simulink model "DatcomForceMoment"  (Simulink 8.8)
settings: Solver=FixedStepDiscrete  StartTime=0.0  StopTime=0.1  FixedStep=.1  RelTol=1e-3
values from neighbouring files (symbols this model uses):
  nfs = PlaneData('SI')    [AFDSimInit.m]    (also in AFDSimInitDatcom.m; TransferFunction.m = PlaneData('Imperial'))
undefined symbols (not defined in the file or in its folder): datcom, Newton, Raphson, sigbuilder_block
libraries: aerolibutil x12, aerolibtransform2 x1, aerolibasang x1
(part 1 of 2)
settings Model: Creator=AHKh  LastModifiedBy=AHKh
settings DataIOCC: LimitDataPoints=off  SaveFormat=Dataset  SignalLoggingSaveFormat=Dataset  SignalLogging=off  DSMLogging=off  SaveTime=off
settings OptimizationCC: LifeSpan=auto
settings DebuggingCC: UnderspecifiedInitializationDetection=Simplified  MergeDetectMultiDrivingBlocksExec=error  FcnCallInpInsideContextMsg=error  StateNameClashWarn=none  SFUnexpectedBacktrackingDiag=error  SFNoUnconditionalDefaultTransitionDiag=error  SFExecutionAtInitializationDiag=warning
settings HardwareCC: ProdBitPerPointer=64  ProdBitPerSizeT=64  ProdBitPerPtrDiffT=64  ProdLargestAtomicFloat=Float  ProdIntDivRoundTo=Zero  ProdEndianess=LittleEndian  ProdWordSize=64  ProdHWDeviceType=Intel->x86-64 (Windows64)
settings ModelReferenceCC: PropagateSignalLabelsOutOfModel=on
settings GRTTargetCC: TargetLangStandard=C99 (ISO)  GeneratePreprocessorConditionals=Use local settings  CombineOutputUpdateFcns=on  GRTInterface=off
settings ConfigComp: CovMetricSettings=dwe  CovHtmlReporting=off  CovSaveCumulativeToWorkspaceVar=off  CovSaveSingleToWorkspaceVar=off  CovExternalEMLEnable=on

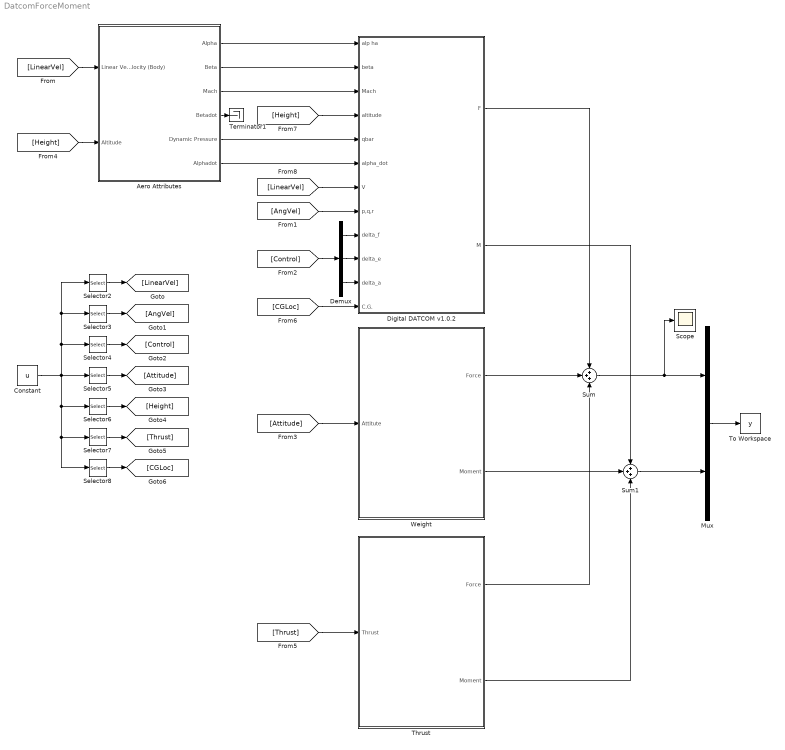
== system DatcomForceMoment ==
  Aero Attributes : Subsystem
  Constant : Constant  Value=u
  Demux : Demux  Outputs=3
  Digital DATCOM v1.0.2 : Subsystem  mask(DATCOM Aerodynamic Forces and Moments Estimation){datcom=datcom}
      mask prompts: datcom "Datcom Structure"
      mask Display:
      | port_label('input',1,'\alpha (rad)','texmode','on');
      | port_label('input',2,'\beta (rad)','texmode','on');
      | port_label('input',3,'Mach','texmode','on');
      | port_label('input',4,'h (m)','texmode','on');
      | port_label('input',5,'q_{bar}','texmode','on');
      | port_label('input',6,'d\alpha/dt (rad/s)','texmode','on');
      | port_label('input',7,'V_{body} m/s','texmode','on');
      | port_label('input',8,'\omega (rad/s)','texmode','on');
      | port_label('input',9,'\delta_F (rad)','texmode','on');
      | port_label('input',10,'\delta_E (rad)','texmode','on');
      | port_label('input',11,'\delta_A (rad)','texmode','on');
      | port_label('input',12,'C.G. (m)','texmode','on');
      | port_label('output',1,'F_{body} (N)','texmode','on');
      | port_label('output',2,'M_{body} (N.m)','texmode','on');
  Mux : Mux  Inputs=2
  Scope : Scope
  Selector2 : Selector  InputPortWidth=17  IndexOptions=Index vector (dialog)  Indices=[1:3]  OutputSizes=1
  Selector3 : Selector  InputPortWidth=17  IndexOptions=Index vector (dialog)  Indices=[4:6]  OutputSizes=1
  Selector4 : Selector  InputPortWidth=17  IndexOptions=Index vector (dialog)  Indices=[7:9]  OutputSizes=1
  Selector5 : Selector  InputPortWidth=17  IndexOptions=Index vector (dialog)  Indices=[10:12]  OutputSizes=1
  Selector6 : Selector  InputPortWidth=17  IndexOptions=Index vector (dialog)  Indices=[13]  OutputSizes=1
  Selector7 : Selector  InputPortWidth=17  IndexOptions=Index vector (dialog)  Indices=[14]  OutputSizes=1
  Selector8 : Selector  InputPortWidth=17  IndexOptions=Index vector (dialog)  Indices=[15:17]  OutputSizes=1
  Sum : Sum  Inputs=+++
  Sum1 : Sum  Inputs=+++
  Terminator1 : Terminator
  "Thrust " : Subsystem
  To Workspace : ToWorkspace  VariableName=y  SampleTime=-1
  Weight : Subsystem
  wires:
  [Height] -> Aero Attributes/2(Altitude)
  [LinearVel] -> Aero Attributes/1(Linear Velocity (Body))
  Aero Attributes/4(Betadot) -> Terminator1/1
  [AngVel] -> Digital DATCOM v1.0.2/8(p,q,r)
  [Height] -> Digital DATCOM v1.0.2/4(altitude)
  [Control] -> Demux/1
  Demux/1 -> Digital DATCOM v1.0.2/9(delta_f)
  Demux/2 -> Digital DATCOM v1.0.2/10(delta_e)
  Demux/3 -> Digital DATCOM v1.0.2/11(delta_a)
  [LinearVel] -> Digital DATCOM v1.0.2/7(V)
  Aero Attributes/1(Alpha) -> Digital DATCOM v1.0.2/1(alp ha)
  Aero Attributes/2(Beta) -> Digital DATCOM v1.0.2/2(beta)
  Aero Attributes/5(Dynamic Pressure) -> Digital DATCOM v1.0.2/5(qbar)
  Aero Attributes/3(Mach) -> Digital DATCOM v1.0.2/3(Mach)
  Aero Attributes/6(Alphadot) -> Digital DATCOM v1.0.2/6(alpha_dot)
  [Attitude] -> Weight/1(Attitute)
  Digital DATCOM v1.0.2/1(F) -> Sum/1
  Weight/1(Force) -> Sum/2
  "Thrust "/1(Force) -> Sum/3
  Sum/1 -> Scope/1, Mux/1
  Weight/2(Moment) -> Sum1/2
  Digital DATCOM v1.0.2/2(M) -> Sum1/1
  "Thrust "/2(Moment) -> Sum1/3
  Sum1/1 -> Mux/2
  [CGLoc] -> Digital DATCOM v1.0.2/12(C.G.)
  [Thrust] -> "Thrust "/1(Thrust)
  Constant/1 -> Selector6/1, Selector8/1, Selector7/1, Selector2/1, Selector3/1, Selector4/1, Selector5/1
  Selector2/1 -> [LinearVel]
  Selector3/1 -> [AngVel]
  Selector4/1 -> [Control]
  Selector5/1 -> [Attitude]
  Selector6/1 -> [Height]
  Selector7/1 -> [Thrust]
  Selector8/1 -> [CGLoc]
  Mux/1 -> To Workspace/1

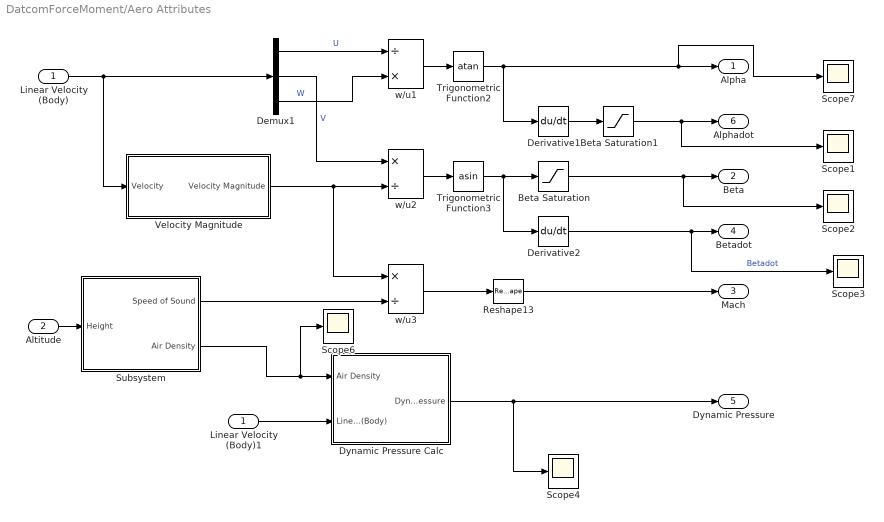
== system DatcomForceMoment/Aero Attributes ==
  Linear Velocity (Body) : Inport  PortDimensions=[3,1]
  Altitude : Inport  Port=2
  Beta Saturation : Saturate  UpperLimit=5*pi/11  LowerLimit=-5*pi/11
  Beta Saturation1 : Saturate  UpperLimit=1  LowerLimit=-1
  Demux1 : Demux  Outputs=3
  Derivative1 : Derivative
  Derivative2 : Derivative
  Dynamic Pressure Calc : Subsystem
  Linear Velocity (Body)1 : InportShadow  PortDimensions=[3,1]
  Reshape13 : Reshape
  Scope{1..4,6..7} (6 alike) : Scope
  Subsystem : Subsystem
  Trigonometric Function2 : Trigonometry  Operator=atan
  Trigonometric Function3 : Trigonometry  Operator=asin
  Velocity Magnitude : Subsystem
  w/u1 : Product  Inputs=/*  SaturateOnIntegerOverflow=on  InputSameDT=on  OutDataTypeStr=Inherit: Same as first input
  w/u2 : Product  Inputs=*/  SaturateOnIntegerOverflow=on  InputSameDT=on  OutDataTypeStr=Inherit: Same as first input
  w/u3 : Product  Inputs=*/  SaturateOnIntegerOverflow=on  InputSameDT=on  OutDataTypeStr=Inherit: Same as first input
  Alpha : Outport
  Beta : Outport  Port=2
  Mach : Outport  Port=3
  Betadot : Outport  Port=4
  Dynamic Pressure : Outport  Port=5
  Alphadot : Outport  Port=6
  wires:
  Beta Saturation1/1 -> Alphadot/1, Scope1/1
  Subsystem/2(Air Density) -> Scope6/1, Dynamic Pressure Calc/1(Air Density)
  Subsystem/1(Speed of Sound) -> w/u3/2
  Velocity Magnitude/1(Velocity Magnitude) -> w/u3/1, w/u2/2
  Reshape13/1 -> Mach/1
  Derivative2/1 -> Betadot/1, Scope3/1  "Betadot"
  Beta Saturation/1 -> Beta/1, Scope2/1
  Derivative1/1 -> Beta Saturation1/1
  Dynamic Pressure Calc/1(Dynamic Pressure) -> Scope4/1, Dynamic Pressure/1
  Linear Velocity (Body)1/1 -> Dynamic Pressure Calc/2(Linear Velocity (Body))
  Altitude/1 -> Subsystem/1(Height)
  w/u3/1 -> Reshape13/1
  Trigonometric Function3/1 -> Beta Saturation/1, Derivative2/1
  Trigonometric Function2/1 -> Derivative1/1, Alpha/1, Scope7/1
  w/u2/1 -> Trigonometric Function3/1
  w/u1/1 -> Trigonometric Function2/1
  Demux1/3 -> w/u1/2  "W"
  Demux1/2 -> w/u2/1  "V"
  Demux1/1 -> w/u1/1  "U"
  Linear Velocity (Body)/1 -> Velocity Magnitude/1(Velocity), Demux1/1

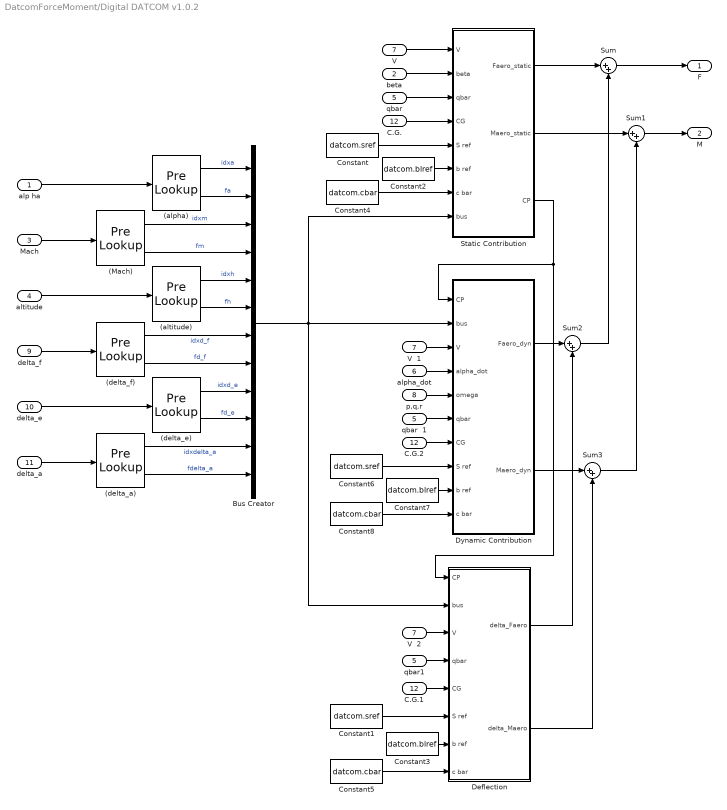
== system DatcomForceMoment/Digital DATCOM v1.0.2 ==
  alp ha : Inport  Unit=rad
  beta : Inport  Port=2  Unit=rad
  Mach : Inport  Port=3  Unit=1
  altitude : Inport  Port=4  Unit=m
  qbar : Inport  Port=5  Unit=Pa
  alpha_dot : Inport  Port=6  Unit=rad/s
  V : Inport  Port=7  Unit=m/s
  p,q,r : Inport  Port=8  Unit=rad/s
  delta_f : Inport  Port=9  Unit=rad
  delta_e : Inport  Port=10  Unit=rad
  delta_a : Inport  Port=11  Unit=rad
  C.G. : Inport  Port=12  Unit=m
  (Mach) : PreLookup  BreakpointsData=datcom.mach  BeginIndexSearchUsingPreviousIndexResult=on  IndexDataTypeStr=int32  FractionDataTypeStr=double
  (alpha) : PreLookup  BreakpointsData=datcom.alpha  BeginIndexSearchUsingPreviousIndexResult=on  IndexDataTypeStr=int32  FractionDataTypeStr=double
  (altitude) : PreLookup  BreakpointsData=datcom.alt  BeginIndexSearchUsingPreviousIndexResult=on  IndexDataTypeStr=int32  FractionDataTypeStr=double
  (delta_a) : PreLookup  BreakpointsData=datcom.deltal-datcom.deltar  BeginIndexSearchUsingPreviousIndexResult=on  IndexDataTypeStr=int32  FractionDataTypeStr=double
  (delta_e) : PreLookup  BreakpointsData=datcom.delta  BeginIndexSearchUsingPreviousIndexResult=on  IndexDataTypeStr=int32  FractionDataTypeStr=double
  (delta_f) : PreLookup  BreakpointsData=datcom.delta  BeginIndexSearchUsingPreviousIndexResult=on  IndexDataTypeStr=int32  FractionDataTypeStr=double
  Bus Creator : BusCreator  Inputs=12
  C.G.1 : InportShadow  Port=12  Unit=m
  C.G.2 : InportShadow  Port=12  Unit=m
  Constant : Constant  Value=datcom.sref
  Constant1 : Constant  Value=datcom.sref
  Constant2 : Constant  Value=datcom.blref
  Constant3 : Constant  Value=datcom.blref
  Constant4 : Constant  Value=datcom.cbar
  Constant5 : Constant  Value=datcom.cbar
  Constant6 : Constant  Value=datcom.sref
  Constant7 : Constant  Value=datcom.blref
  Constant8 : Constant  Value=datcom.cbar
  Deflection : Subsystem
  Dynamic Contribution : Subsystem
  Static Contribution : Subsystem
  Sum{,1..3} (4 alike) : Sum  Inputs=|++
  V  1 : InportShadow  Port=7  Unit=m/s
  V  2 : InportShadow  Port=7  Unit=m/s
  qbar  1 : InportShadow  Port=5  Unit=Pa
  qbar1 : InportShadow  Port=5  Unit=Pa
  F : Outport  Unit=N
  M : Outport  Port=2  Unit=N*m
  wires:
  Constant8/1 -> Dynamic Contribution/10(c bar)
  Constant6/1 -> Dynamic Contribution/8(S ref)
  Constant7/1 -> Dynamic Contribution/9(b ref)
  C.G.2/1 -> Dynamic Contribution/7(CG)
  Constant4/1 -> Static Contribution/7(c bar)
  Constant5/1 -> Deflection/8(c bar)
  Constant3/1 -> Deflection/7(b ref)
  Constant2/1 -> Static Contribution/6(b ref)
  Constant1/1 -> Deflection/6(S ref)
  Constant/1 -> Static Contribution/5(S ref)
  C.G.1/1 -> Deflection/5(CG)
  C.G./1 -> Static Contribution/4(CG)
  Deflection/2(delta_Maero) -> Sum3/2
  Deflection/1(delta_Faero) -> Sum2/2
  Sum3/1 -> Sum1/2
  Sum2/1 -> Sum/2
  qbar1/1 -> Deflection/4(qbar)
  V  2/1 -> Deflection/3("V ")
  (delta_a)/2 -> Bus Creator/12  "fdelta_a"
  (delta_a)/1 -> Bus Creator/11  "idxdelta_a"
  (delta_e)/2 -> Bus Creator/10  "fd_e"
  (delta_e)/1 -> Bus Creator/9  "idxd_e"
  V/1 -> Static Contribution/1("V ")
  V  1/1 -> Dynamic Contribution/3(V)
  qbar/1 -> Static Contribution/3(qbar)
  beta/1 -> Static Contribution/2(beta)
  (alpha)/2 -> Bus Creator/2  "fa"
  (Mach)/2 -> Bus Creator/4  "fm"
  (altitude)/2 -> Bus Creator/6  "fh"
  (altitude)/1 -> Bus Creator/5  "idxh"
  (delta_f)/2 -> Bus Creator/8  "fd_f"
  (delta_f)/1 -> Bus Creator/7  "idxd_f"
  qbar  1/1 -> Dynamic Contribution/6(qbar)
  p,q,r/1 -> Dynamic Contribution/5(omega)
  alpha_dot/1 -> Dynamic Contribution/4(alpha_dot)
  Sum1/1 -> M/1
  Sum/1 -> F/1
  Dynamic Contribution/2(Maero_dyn) -> Sum3/1
  Static Contribution/2(Maero_static) -> Sum1/1
  Dynamic Contribution/1(Faero_dyn) -> Sum2/1
  Static Contribution/1(Faero_static) -> Sum/1
  Static Contribution/3("CP ") -> Deflection/1(CP), Dynamic Contribution/1(CP)
  (Mach)/1 -> Bus Creator/3  "idxm"
  (alpha)/1 -> Bus Creator/1  "idxa"
  Bus Creator/1 -> Deflection/2(bus), Dynamic Contribution/2(bus), Static Contribution/8(bus)
  alp ha/1 -> (alpha)/1
  Mach/1 -> (Mach)/1
  altitude/1 -> (altitude)/1
  delta_f/1 -> (delta_f)/1
  delta_e/1 -> (delta_e)/1
  delta_a/1 -> (delta_a)/1

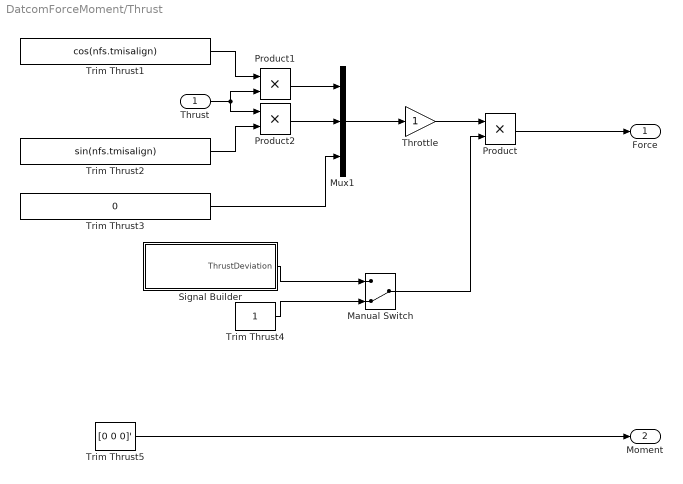
== system DatcomForceMoment/Thrust  ==
  Thrust : Inport  PortDimensions=[1,1]
  Manual Switch : ManualSwitch  CurrentSetting=0
  Mux1 : Mux  Inputs=3
  Product : Product  RndMeth=Zero
  Product1 : Product  RndMeth=Zero
  Product2 : Product  RndMeth=Zero
  Signal Builder : Subsystem  Tag=STV Subsys  LoadFcn=sigbuilder_block('load');  StartFcn=sigbuilder_block('start');  StopFcn=sigbuilder_block('stop');  ClipboardFcn=sigbuilder_block('clipboard');  mask(Sigbuilder block){tuvar=[0:10]}
      mask help: Simulink:masks:SigbuilderBlock_MD
      mask init:
      | if ~strcmp(get_param(bdroot(gcbh),'SimulationStatus'),'stopped') tuvar = sigbuilder_block('maskInit'); end
      settings: CopyFcn=sigbuilder_block('copy');  DeleteFcn=sigbuilder_block('delete');  ModelCloseFcn=sigbuilder_block('modelClose');  PreSaveFcn=sigbuilder_block('preSave');  PauseFcn=sigbuilder_block('pause');  ContinueFcn=sigbuilder_block('continue');  NameChangeFcn=sigbuilder_block('namechange');  OpenFcn=sigbuilder_block('open',[437.4 199.2 550.2 400.2 ]);  CloseFcn=sigbuilder_block('close');
      mask Display: plot(0, 0, 100, 100,[2, 2, 32, 32, 2], [68, 8, 8, 68, 68],[32, 2], [38, 38], [32, 19, 2],[53, 60, 44], [32, 17, 17, 2],[16, 16, 31, 31]);txt = getActiveGroup(gcbh);text(2, 100, txt,'verticalAlignment', 'top');
  Throttle : Gain
  Trim Thrust1 : Constant  Value=cos(nfs.tmisalign)
  Trim Thrust2 : Constant  Value=sin(nfs.tmisalign)
  Trim Thrust3 : Constant  Value=0
  Trim Thrust4 : Constant
  Trim Thrust5 : Constant  Value=[0 0 0]'
  Force : Outport  Unit=N  PortDimensions=[3,1]
  Moment : Outport  Port=2  Unit=N*m  PortDimensions=[3,1]
  wires:
  Mux1/1 -> Throttle/1
  Trim Thrust3/1 -> Mux1/3
  Throttle/1 -> Product/1
  Product/1 -> Force/1
  Manual Switch/1 -> Product/2
  Signal Builder/1(ThrustDeviation) -> Manual Switch/1
  Trim Thrust4/1 -> Manual Switch/2
  Trim Thrust5/1 -> Moment/1
  Trim Thrust1/1 -> Product1/1
  Thrust/1 -> Product2/1, Product1/2
  Product2/1 -> Mux1/2
  Product1/1 -> Mux1/1
  Trim Thrust2/1 -> Product2/2

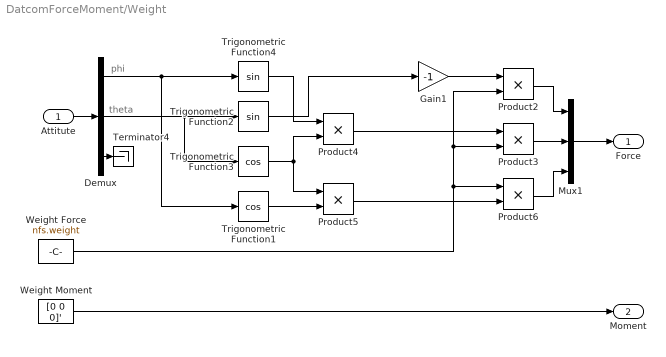
== system DatcomForceMoment/Weight ==
  note: theta
  note: phi
  Attitute : Inport  PortDimensions=[3,1]
  Demux : Demux  Outputs=3
  Gain1 : Gain  Gain=-1
  Mux1 : Mux  Inputs=3
  Product{2..6} (5 alike) : Product  RndMeth=Zero
  Terminator4 : Terminator
  Trigonometric Function1 : Trigonometry  Operator=cos
  Trigonometric Function2 : Trigonometry
  Trigonometric Function3 : Trigonometry  Operator=cos
  Trigonometric Function4 : Trigonometry
  Weight Force : Constant  Value=nfs.weight
  Weight Moment : Constant  Value=[0 0 0]'
  Force : Outport  Unit=N  PortDimensions=[3,1]
  Moment : Outport  Port=2  Unit=N*m  PortDimensions=[3,1]
  wires:
  Mux1/1 -> Force/1
  Product6/1 -> Mux1/3
  Product3/1 -> Mux1/2
  Product2/1 -> Mux1/1
  Product5/1 -> Product6/2
  Product4/1 -> Product3/1
  Trigonometric Function1/1 -> Product5/2
  Trigonometric Function4/1 -> Product4/1
  Trigonometric Function3/1 -> Product5/1, Product4/2
  Trigonometric Function2/1 -> Gain1/1
  Weight Force/1 -> Product6/1, Product3/2, Product2/2
  Gain1/1 -> Product2/1
  Demux/3 -> Terminator4/1
  Attitute/1 -> Demux/1
  Demux/2 -> Trigonometric Function3/1, Trigonometric Function2/1
  Demux/1 -> Trigonometric Function1/1, Trigonometric Function4/1
  Weight Moment/1 -> Moment/1

== system DatcomForceMoment/Aero Attributes/Dynamic Pressure Calc ==
  Air Density : Inport  PortDimensions=1
  Linear Velocity (Body) : Inport  Port=2  PortDimensions=[3 1]
  0.5*rh : Product  SaturateOnIntegerOverflow=on  InputSameDT=on  OutDataTypeStr=Inherit: Same as first input
  Dot Product : DotProduct  InputSameDT=on  OutDataTypeStr=Inherit: Inherit via internal rule
  Gain : Gain  Gain=0.5  SaturateOnIntegerOverflow=on  OutDataTypeStr=Inherit: Same as input  ParamDataTypeStr=Inherit: Same as input
  V^2 : Abs
  Dynamic Pressure : Outport
  wires:
  Dot Product/1 -> V^2/1
  Linear Velocity (Body)/1 -> Dot Product/2, Dot Product/1
  Air Density/1 -> Gain/1
  V^2/1 -> 0.5*rh/1
  Gain/1 -> 0.5*rh/2
  0.5*rh/1 -> Dynamic Pressure/1

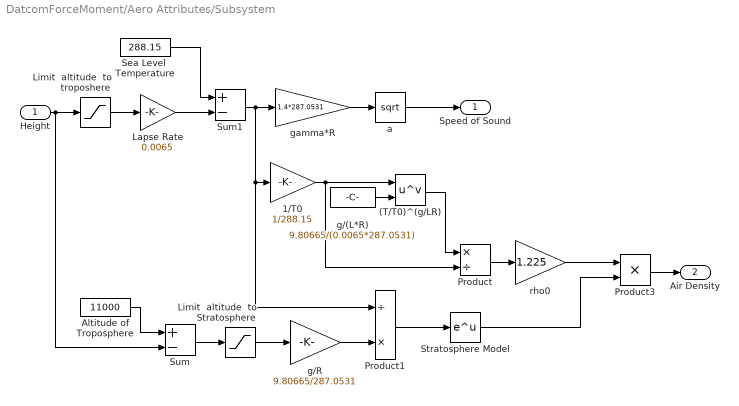
== system DatcomForceMoment/Aero Attributes/Subsystem ==
  Height : Inport
  "(T/T0)^(g/LR) " : Math  Operator=pow  SaturateOnIntegerOverflow=on
  1/T0 : Gain  Gain=1/288.15  SaturateOnIntegerOverflow=on  OutDataTypeStr=Inherit: Same as input  ParamDataTypeStr=Inherit: Same as input
  Altitude of Troposphere : Constant  Value=11000  OutDataTypeStr=Inherit: Inherit via back propagation
  Lapse Rate : Gain  Gain=0.0065  SaturateOnIntegerOverflow=on  OutDataTypeStr=Inherit: Same as input  ParamDataTypeStr=Inherit: Same as input
  Limit  altitude  to Stratosphere : Saturate  UpperLimit=0  LowerLimit=11000-20000
  Limit  altitude  to troposhere : Saturate  UpperLimit=11000  LowerLimit=0
  Product : Product  Inputs=*/  SaturateOnIntegerOverflow=on  InputSameDT=on  OutDataTypeStr=Inherit: Same as first input
  Product1 : Product  Inputs=/*  SaturateOnIntegerOverflow=on  InputSameDT=on  OutDataTypeStr=Inherit: Same as first input
  Product3 : Product  SaturateOnIntegerOverflow=on  InputSameDT=on  OutDataTypeStr=Inherit: Same as first input
  Sea Level  Temperature : Constant  Value=288.15  OutDataTypeStr=Inherit: Inherit via back propagation
  Stratosphere Model : Math  SaturateOnIntegerOverflow=on
  Sum : Sum  Inputs=+-  SaturateOnIntegerOverflow=on  InputSameDT=on  OutDataTypeStr=Inherit: Same as first input
  Sum1 : Sum  Inputs=+-  SaturateOnIntegerOverflow=on  InputSameDT=on  OutDataTypeStr=Inherit: Same as first input
  a : Sqrt  AlgorithmType=Newton-Raphson  SaturateOnIntegerOverflow=on
  g/(L*R) : Constant  Value=9.80665/(0.0065*287.0531)  OutDataTypeStr=Inherit: Inherit via back propagation
  g/R : Gain  Gain=9.80665/287.0531  SaturateOnIntegerOverflow=on  OutDataTypeStr=Inherit: Same as input  ParamDataTypeStr=Inherit: Same as input
  gamma*R : Gain  Gain=1.4*287.0531  SaturateOnIntegerOverflow=on  OutDataTypeStr=Inherit: Same as input  ParamDataTypeStr=Inherit: Same as input
  rho0 : Gain  Gain=1.225  SaturateOnIntegerOverflow=on  OutDataTypeStr=Inherit: Same as input  ParamDataTypeStr=Inherit: Same as input
  Speed of Sound : Outport  PortDimensions=1
  Air Density : Outport  Port=2  PortDimensions=1
  wires:
  g/(L*R)/1 -> "(T/T0)^(g/LR) "/2
  Height/1 -> Limit  altitude  to troposhere/1, Sum/2
  Limit  altitude  to troposhere/1 -> Lapse Rate/1
  Product/1 -> rho0/1
  "(T/T0)^(g/LR) "/1 -> Product/1
  1/T0/1 -> "(T/T0)^(g/LR) "/1, Product/2
  gamma*R/1 -> a/1
  a/1 -> Speed of Sound/1
  Sum1/1 -> gamma*R/1, 1/T0/1, Product1/1
  Lapse Rate/1 -> Sum1/2
  Sea Level  Temperature/1 -> Sum1/1
  rho0/1 -> Product3/1
  Product3/1 -> Air Density/1
  Stratosphere Model/1 -> Product3/2
  g/R/1 -> Product1/2
  Product1/1 -> Stratosphere Model/1
  Altitude of Troposphere/1 -> Sum/1
  Sum/1 -> Limit  altitude  to Stratosphere/1
  Limit  altitude  to Stratosphere/1 -> g/R/1

== system DatcomForceMoment/Aero Attributes/Velocity Magnitude ==
  Velocity : Inport
  Dot Product : DotProduct  InputSameDT=on  OutDataTypeStr=Inherit: Inherit via internal rule
  Sqrt : Sqrt  SaturateOnIntegerOverflow=on
  Velocity Magnitude : Outport
  wires:
  Sqrt/1 -> Velocity Magnitude/1  "abs(V)"
  Velocity/1 -> Dot Product/2, Dot Product/1
  Dot Product/1 -> Sqrt/1

== system DatcomForceMoment/Digital DATCOM v1.0.2/Deflection ==
  CP : Inport
  bus : Inport  Port=2
  "V " : Inport  Port=3
  qbar : Inport  Port=4
  CG : Inport  Port=5
  S ref : Inport  Port=6  Unit=m^2
  b ref : Inport  Port=7  Unit=m  PortDimensions=1
  c bar : Inport  Port=8  Unit=m  PortDimensions=1
  Aerodynamic Forces and Moments : Subsystem
  Delta Coefficients : Subsystem
  delta_Faero : Outport
  delta_Maero : Outport  Port=2
  wires:
  Aerodynamic Forces and Moments/1(Forces) -> delta_Faero/1
  Aerodynamic Forces and Moments/2(Moments) -> delta_Maero/1
  S ref/1 -> Aerodynamic Forces and Moments/6(S ref)
  b ref/1 -> Aerodynamic Forces and Moments/7(b ref)
  qbar/1 -> Aerodynamic Forces and Moments/2(qbar)
  c bar/1 -> Aerodynamic Forces and Moments/8(cbar)
  CG/1 -> Aerodynamic Forces and Moments/3(CG)
  "V "/1 -> Aerodynamic Forces and Moments/5(Vb)
  CP/1 -> Aerodynamic Forces and Moments/4(CP)
  Delta Coefficients/1(delCoeff) -> Aerodynamic Forces and Moments/1(Coefficients)
  bus/1 -> Delta Coefficients/1(bus)

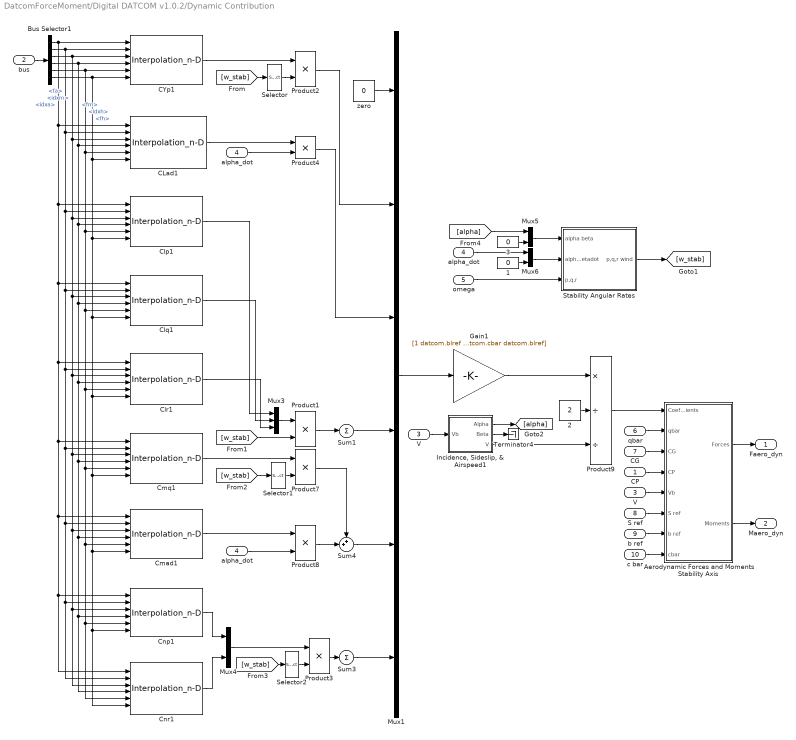
== system DatcomForceMoment/Digital DATCOM v1.0.2/Dynamic Contribution ==
  CP : Inport
  bus : Inport  Port=2
  V : Inport  Port=3
  alpha_dot : Inport  Port=4  Unit=rad/s
  omega : Inport  Port=5  Unit=rad/s
  qbar : Inport  Port=6
  CG : Inport  Port=7
  S ref : Inport  Port=8  Unit=m^2
  b ref : Inport  Port=9  Unit=m  PortDimensions=1
  c bar : Inport  Port=10  Unit=m  PortDimensions=1
  " V " : InportShadow  Port=3
  " alpha_dot " : InportShadow  Port=4  Unit=rad/s
  1 : Constant  Value=0
  2 : Constant  Value=2
  3 : Constant  Value=0
  Aerodynamic Forces and Moments Stability Axis : Subsystem
  Bus Selector1 : BusSelector  OutputSignals=idxa,fa,idxm,fm,idxh,fh
  CLad1 : Interpolation_n-D  NumberOfTableDimensions=3  Table="permute(datcom.clad,[1  2  3])"  OutDataTypeStr=double
      settings: InputPortMap=u0,u1,u2,u3,u4,u5
  CYp1 : Interpolation_n-D  NumberOfTableDimensions=3  Table="permute(datcom.cyp,[1  2  3])"  OutDataTypeStr=double
      settings: InputPortMap=u0,u1,u2,u3,u4,u5
  Clp1 : Interpolation_n-D  NumberOfTableDimensions=3  Table="permute(datcom.clp,[1  2  3])"  OutDataTypeStr=double
      settings: InputPortMap=u0,u1,u2,u3,u4,u5
  Clq1 : Interpolation_n-D  NumberOfTableDimensions=3  Table="permute(datcom.clq,[1  2  3])"  OutDataTypeStr=double
      settings: InputPortMap=u0,u1,u2,u3,u4,u5
  Clr1 : Interpolation_n-D  NumberOfTableDimensions=3  Table="permute(datcom.clr,[1  2  3])"  OutDataTypeStr=double
      settings: InputPortMap=u0,u1,u2,u3,u4,u5
  Cmad1 : Interpolation_n-D  NumberOfTableDimensions=3  Table="permute(datcom.cmad,[1  2  3])"  OutDataTypeStr=double
      settings: InputPortMap=u0,u1,u2,u3,u4,u5
  Cmq1 : Interpolation_n-D  NumberOfTableDimensions=3  Table="permute(datcom.cmq,[1  2  3])"  OutDataTypeStr=double
      settings: InputPortMap=u0,u1,u2,u3,u4,u5
  Cnp1 : Interpolation_n-D  NumberOfTableDimensions=3  Table="permute(datcom.cnp,[1  2  3])"  OutDataTypeStr=double
      settings: InputPortMap=u0,u1,u2,u3,u4,u5
  Cnr1 : Interpolation_n-D  NumberOfTableDimensions=3  Table="permute(datcom.cnr,[1  2  3])"  OutDataTypeStr=double
      settings: InputPortMap=u0,u1,u2,u3,u4,u5
  Gain1 : Gain  Gain=[1 datcom.blref datcom.cbar datcom.blref datcom.cbar datcom.blref]
  "Incidence, Sideslip, & Airspeed1" : Subsystem
      mask Display:
      | port_label('input',1,'V_b','texmode','on');
      | port_label('output',1,'\alpha','texmode','on');
      | port_label('output',2,'\beta','texmode','on');
      | port_label('output',3,'V','texmode','on');
  Mux1 : Mux  Inputs=6
  Mux3 : Mux  Inputs=3
  Mux4 : Mux  Inputs=2
  Mux5 : Mux  Inputs=2
  Mux6 : Mux  Inputs=2
  Product{1..4,7..8} (6 alike) : Product  RndMeth=Zero
  Product9 : Product  Inputs=*//  RndMeth=Zero
  Selector : Selector  InputPortWidth=3  IndexOptions=Index vector (dialog)  Indices=1  OutputSizes=1
  Selector1 : Selector  InputPortWidth=3  IndexOptions=Index vector (dialog)  Indices=2  OutputSizes=1
  Selector2 : Selector  InputPortWidth=3  IndexOptions=Index vector (dialog)  Indices=[1 3]  OutputSizes=1
  Stability Angular Rates : Subsystem
      mask Display:
      | port_label('input',1,'\alpha \beta','texmode','on');
      | port_label('input',2,'d\alpha/dt d\beta/dt','texmode','on');
      | port_label('input',3,'\omega','texmode','on');
      | port_label('output',1,'\omega_w','texmode','on');
  Sum1 : Sum  Inputs=+
  Sum3 : Sum  Inputs=+
  Sum4 : Sum  Inputs=++|
  Terminator4 : Terminator
  "alpha_dot " : InportShadow  Port=4  Unit=rad/s
  zero : Constant  Value=0
  Faero_dyn : Outport
  Maero_dyn : Outport  Port=2
  wires:
  c bar/1 -> Aerodynamic Forces and Moments Stability Axis/8(cbar)
  b ref/1 -> Aerodynamic Forces and Moments Stability Axis/7(b ref)
  S ref/1 -> Aerodynamic Forces and Moments Stability Axis/6(S ref)
  CLad1/1 -> Product4/1
  Bus Selector1/6 -> Clp1/6, Clq1/6, Clr1/6, Cmq1/6, Cmad1/6, Cnp1/6, Cnr1/6, CLad1/6, CYp1/6  "<fh>"
  Bus Selector1/5 -> Clp1/5, Clq1/5, Clr1/5, Cmq1/5, Cmad1/5, Cnp1/5, Cnr1/5, CLad1/5, CYp1/5  "<idxh>"
  Bus Selector1/4 -> Clp1/4, Clq1/4, Clr1/4, Cmq1/4, Cmad1/4, Cnp1/4, Cnr1/4, CLad1/4, CYp1/4  "<fm>"
  Bus Selector1/3 -> Clp1/3, Clq1/3, Clr1/3, Cmq1/3, Cmad1/3, Cnp1/3, Cnr1/3, CLad1/3, CYp1/3  "<idxm>"
  Bus Selector1/2 -> Clp1/2, Clq1/2, Clr1/2, Cmq1/2, Cmad1/2, Cnp1/2, Cnr1/2, CLad1/2, CYp1/2  "<fa>"
  Bus Selector1/1 -> Clp1/1, Clq1/1, Clr1/1, Cmq1/1, Cmad1/1, Cnp1/1, Cnr1/1, CLad1/1, CYp1/1  "<idxa>"
  bus/1 -> Bus Selector1/1
  " alpha_dot "/1 -> Mux6/1
  omega/1 -> Stability Angular Rates/3(p,q,r)
  Stability Angular Rates/1(p,q,r wind) -> [w_stab]
  Mux1/1 -> Gain1/1
  Cnp1/1 -> Mux4/1
  Cmq1/1 -> Product7/1
  Sum1/1 -> Mux1/4
  Product2/1 -> Mux1/2
  Clq1/1 -> Mux3/2
  Selector/1 -> Product2/2
  CYp1/1 -> Product2/1
  "alpha_dot "/1 -> Product4/2
  [w_stab] -> Selector/1
  Clr1/1 -> Mux3/3
  Clp1/1 -> Mux3/1
  Mux3/1 -> Product1/1
  [w_stab] -> Product1/2
  Product1/1 -> Sum1/1
  [w_stab] -> Selector1/1
  Selector1/1 -> Product7/2
  Product7/1 -> Sum4/1
  Cmad1/1 -> Product8/1
  Product8/1 -> Sum4/2
  alpha_dot/1 -> Product8/2
  Cnr1/1 -> Mux4/2
  [w_stab] -> Selector2/1
  Mux4/1 -> Product3/1
  Selector2/1 -> Product3/2
  Sum3/1 -> Mux1/6
  Product3/1 -> Sum3/1
  Gain1/1 -> Product9/1
  Product9/1 -> Aerodynamic Forces and Moments Stability Axis/1(Coefficients)
  2/1 -> Product9/2
  V/1 -> "Incidence, Sideslip, & Airspeed1"/1(Vb)
  Sum4/1 -> Mux1/5
  Product4/1 -> Mux1/3
  zero/1 -> Mux1/1
  "Incidence, Sideslip, & Airspeed1"/3(V) -> Product9/3
  "Incidence, Sideslip, & Airspeed1"/2(Beta) -> Terminator4/1
  "Incidence, Sideslip, & Airspeed1"/1(Alpha) -> [alpha]
  Aerodynamic Forces and Moments Stability Axis/1(Forces) -> Faero_dyn/1
  qbar/1 -> Aerodynamic Forces and Moments Stability Axis/2(qbar)
  Aerodynamic Forces and Moments Stability Axis/2(Moments) -> Maero_dyn/1
  " V "/1 -> Aerodynamic Forces and Moments Stability Axis/5(Vb)
  3/1 -> Mux5/2
  [alpha] -> Mux5/1
  Mux5/1 -> Stability Angular Rates/1(alpha beta)
  Mux6/1 -> Stability Angular Rates/2(alphadot betadot)
  1/1 -> Mux6/2
  CG/1 -> Aerodynamic Forces and Moments Stability Axis/3(CG)
  CP/1 -> Aerodynamic Forces and Moments Stability Axis/4(CP)

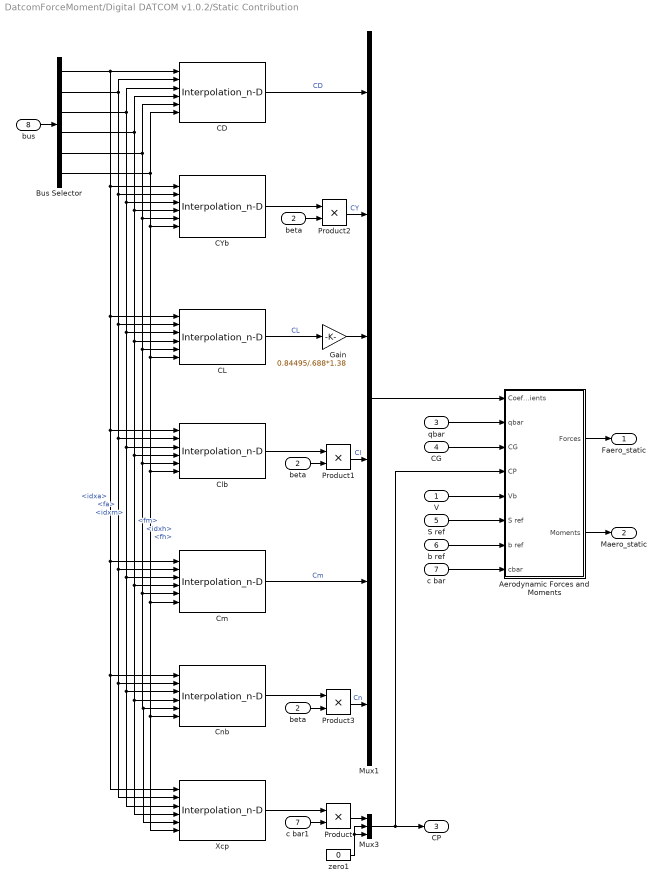
== system DatcomForceMoment/Digital DATCOM v1.0.2/Static Contribution ==
  "V " : Inport
  beta : Inport  Port=2
  qbar : Inport  Port=3
  CG : Inport  Port=4
  S ref : Inport  Port=5  Unit=m^2
  b ref : Inport  Port=6  Unit=m  PortDimensions=1
  c bar : Inport  Port=7  Unit=m  PortDimensions=1
  bus : Inport  Port=8
  " beta " : InportShadow  Port=2
  Aerodynamic Forces and Moments : Subsystem
  Bus Selector : BusSelector  OutputSignals=idxa,fa,idxm,fm,idxh,fh
  CD : Interpolation_n-D  NumberOfTableDimensions=3  Table=permute(datcom.cd,[1 2 3])  InterpMethod=Flat  ExtrapMethod=Clip  OutDataTypeStr=double
      settings: InputPortMap=u0,u1,u2,u3,u4,u5
  CL : Interpolation_n-D  NumberOfTableDimensions=3  Table=permute(datcom.cl,[1 2 3])  InterpMethod=Flat  ExtrapMethod=Clip  OutDataTypeStr=double
      settings: InputPortMap=u0,u1,u2,u3,u4,u5
  CYb : Interpolation_n-D  NumberOfTableDimensions=3  Table=permute(datcom.cyb,[1 2 3])  InterpMethod=Flat  ExtrapMethod=Clip  OutDataTypeStr=double
      settings: InputPortMap=u0,u1,u2,u3,u4,u5
  Clb : Interpolation_n-D  NumberOfTableDimensions=3  Table=permute(datcom.clb,[1 2 3])  InterpMethod=Flat  ExtrapMethod=Clip  OutDataTypeStr=double
      settings: InputPortMap=u0,u1,u2,u3,u4,u5
  Cm : Interpolation_n-D  NumberOfTableDimensions=3  Table=permute(datcom.cm,[1 2 3])  InterpMethod=Flat  ExtrapMethod=Clip  OutDataTypeStr=double
      settings: InputPortMap=u0,u1,u2,u3,u4,u5
  Cnb : Interpolation_n-D  NumberOfTableDimensions=3  Table=permute(datcom.cnb,[1 2 3])  InterpMethod=Flat  ExtrapMethod=Clip  OutDataTypeStr=double
      settings: InputPortMap=u0,u1,u2,u3,u4,u5
  Gain : Gain  Gain=0.84495/.688*1.38
  Mux1 : Mux  Inputs=6
  Mux3 : Mux  Inputs=3
  Product : Product
  Product1 : Product  RndMeth=Zero
  Product2 : Product  RndMeth=Zero
  Product3 : Product  RndMeth=Zero
  Xcp : Interpolation_n-D  NumberOfTableDimensions=3  Table="permute(datcom.xcp,[1  2  3])"  OutDataTypeStr=double
      settings: InputPortMap=u0,u1,u2,u3,u4,u5
  "beta " : InportShadow  Port=2
  c bar1 : InportShadow  Port=7  Unit=m  PortDimensions=1
  zero1 : Constant  Value=0
  Faero_static : Outport
  Maero_static : Outport  Port=2
  "CP " : Outport  Port=3
  wires:
  c bar1/1 -> Product/2
  Product/1 -> Mux3/1
  zero1/1 -> Mux3/3, Mux3/2
  Xcp/1 -> Product/1
  c bar/1 -> Aerodynamic Forces and Moments/8(cbar)
  b ref/1 -> Aerodynamic Forces and Moments/7(b ref)
  S ref/1 -> Aerodynamic Forces and Moments/6(S ref)
  Mux3/1 -> Aerodynamic Forces and Moments/4(CP), "CP "/1
  CG/1 -> Aerodynamic Forces and Moments/3(CG)
  bus/1 -> Bus Selector/1
  Bus Selector/1 -> CD/1, CYb/1, Clb/1, Cnb/1, Xcp/1, Cm/1, CL/1  "<idxa>"
  Bus Selector/2 -> Cnb/2, Xcp/2, Cm/2, Clb/2, CL/2, CYb/2, CD/2  "<fa>"
  Bus Selector/3 -> Cnb/3, Xcp/3, Cm/3, Clb/3, CL/3, CYb/3, CD/3  "<idxm>"
  Bus Selector/4 -> Cnb/4, Xcp/4, Cm/4, Clb/4, CL/4, CYb/4, CD/4  "<fm>"
  Bus Selector/5 -> Cnb/5, Xcp/5, Cm/5, Clb/5, CL/5, CYb/5, CD/5  "<idxh>"
  Bus Selector/6 -> Cnb/6, Xcp/6, Cm/6, Clb/6, CL/6, CYb/6, CD/6  "<fh>"
  CD/1 -> Mux1/1  "CD"
  CL/1 -> Gain/1  "CL"
  CYb/1 -> Product2/1
  beta/1 -> Product2/2
  Clb/1 -> Product1/1
  "beta "/1 -> Product1/2
  Product2/1 -> Mux1/2  "CY"
  Product1/1 -> Mux1/4  "Cl"
  Cm/1 -> Mux1/5  "Cm"
  Cnb/1 -> Product3/1
  " beta "/1 -> Product3/2
  Product3/1 -> Mux1/6  "Cn"
  Mux1/1 -> Aerodynamic Forces and Moments/1(Coefficients)
  Aerodynamic Forces and Moments/1(Forces) -> Faero_static/1
  qbar/1 -> Aerodynamic Forces and Moments/2(qbar)
  Aerodynamic Forces and Moments/2(Moments) -> Maero_static/1
  "V "/1 -> Aerodynamic Forces and Moments/5(Vb)
  Gain/1 -> Mux1/3

== system DatcomForceMoment/Thrust /Signal Builder ==
  Demux : Demux  Tag=STV Demux  Outputs=1
  FromWs : FromWorkspace  Tag=STV FromWs  VariableName=tuvar  SampleTime=0  SigBuilderData=DataTag1  VnvData=DataTag2
      SigBuilderData=|
      | common.afterFinalStr = 'Extrapolate'
      | common.sampleTime = 0
      | dataSet.timeRange = [0 1200]
      | dataSet.name = 'Thrust Deviation'
      | sbobj.Groups.Name = 'Thrust Deviation'
      | sbobj.Groups.Signals.Name = 'ThrustDeviation'
      | sbobj.Groups.Signals.XData = [0 10 10 12 12 1200]
      | sbobj.Groups.Signals.YData = [1 1 1.05 1.05 1 1]
      | sbobj.Groups.TimeRange = [0 1200]
  ThrustDeviation : Outport  Tag=STV Outport
  wires:
  Demux/1 -> ThrustDeviation/1
  FromWs/1 -> Demux/1

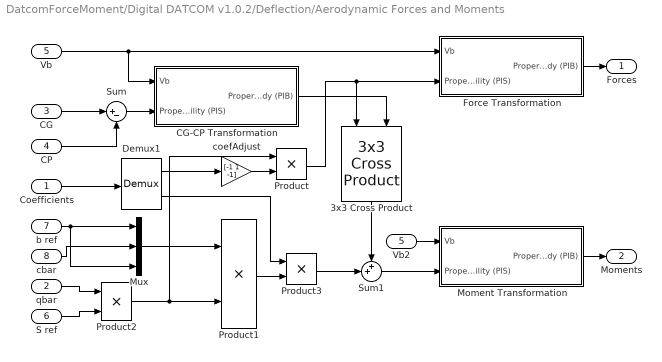
== system DatcomForceMoment/Digital DATCOM v1.0.2/Deflection/Aerodynamic Forces and Moments ==
  Coefficients : Inport
  qbar : Inport  Port=2  Unit=Pa
  CG : Inport  Port=3  Unit=m  PortDimensions=[3, 1]
  CP : Inport  Port=4  Unit=m  PortDimensions=[3,1]
  Vb : Inport  Port=5
  S ref : Inport  Port=6  Unit=m^2  PortDimensions=1
  b ref : Inport  Port=7  Unit=m  PortDimensions=1
  cbar : Inport  Port=8  Unit=m  PortDimensions=1
  3x3 Cross Product : aerolibutil/3x3 Cross Product
  CG-CP Transformation : Subsystem
  Demux1 : Demux  Outputs=[3,3]
  Force Transformation : Subsystem
  Moment Transformation : Subsystem
  Mux : Mux  Inputs=3
  Product{,1..3} (4 alike) : Product  SaturateOnIntegerOverflow=on  InputSameDT=on  OutDataTypeStr=Inherit: Same as first input
  Sum : Sum  Inputs=|+-  SaturateOnIntegerOverflow=on
  Sum1 : Sum  Inputs=++|  SaturateOnIntegerOverflow=on  InputSameDT=on  OutDataTypeStr=Inherit: Same as first input
  Vb2 : InportShadow  Port=5
  coefAdjust : Gain  Gain="[-1  1 -1]"
  Forces : Outport  Unit=N
  Moments : Outport  Port=2  Unit=N
  wires:
  Vb2/1 -> Moment Transformation/1(Vb)
  Sum1/1 -> Moment Transformation/2(Property-In-Stability (PIS))
  S ref/1 -> Product2/2
  Mux/1 -> Product1/1
  b ref/1 -> Mux/3, Mux/1
  cbar/1 -> Mux/2
  3x3 Cross Product/1 -> Sum1/1
  Product1/1 -> Product3/2
  Coefficients/1 -> Demux1/1
  Demux1/2 -> Product3/1
  qbar/1 -> Product2/1
  Product2/1 -> Product1/2, Product/1
  Product3/1 -> Sum1/2
  Demux1/1 -> coefAdjust/1
  Product/1 -> Force Transformation/2(Property-In-Stability (PIS)), 3x3 Cross Product/1
  Force Transformation/1(Property-In-Body (PIB)) -> Forces/1
  Moment Transformation/1(Property-In-Body (PIB)) -> Moments/1
  coefAdjust/1 -> Product/2
  CG/1 -> Sum/1
  CP/1 -> Sum/2
  Sum/1 -> CG-CP Transformation/2(Property-In-Stability (PIS))
  CG-CP Transformation/1(Property-In-Body (PIB)) -> 3x3 Cross Product/2
  Vb/1 -> Force Transformation/1(Vb), CG-CP Transformation/1(Vb)

== system DatcomForceMoment/Digital DATCOM v1.0.2/Deflection/Delta Coefficients ==
  bus : Inport
  Aileron Deflaction : Subsystem
  Elevator Deflaction : Subsystem
  Flap Deflaction : Subsystem
  Gain : Gain  Gain=0
  Sum : Sum  Inputs=+++
  delCoeff : Outport
  wires:
  Sum/1 -> delCoeff/1
  Aileron Deflaction/1(delCoeff_a) -> Gain/1
  Flap Deflaction/1(delCoeff_f) -> Sum/1
  Elevator Deflaction/1(delCoeff_e) -> Sum/2
  bus/1 -> Elevator Deflaction/1(bus), Aileron Deflaction/1(bus), Flap Deflaction/1(bus)
  Gain/1 -> Sum/3

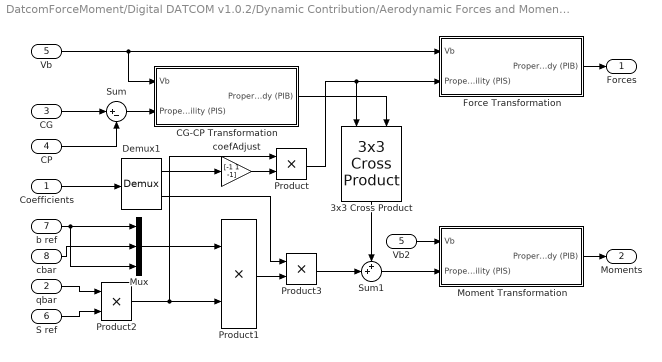
== system DatcomForceMoment/Digital DATCOM v1.0.2/Dynamic Contribution/Aerodynamic Forces and Moments Stability Axis ==
  Coefficients : Inport
  qbar : Inport  Port=2  Unit=Pa
  CG : Inport  Port=3  Unit=m  PortDimensions=[3, 1]
  CP : Inport  Port=4  Unit=m  PortDimensions=[3,1]
  Vb : Inport  Port=5
  S ref : Inport  Port=6  Unit=m^2  PortDimensions=1
  b ref : Inport  Port=7  Unit=m  PortDimensions=1
  cbar : Inport  Port=8  Unit=m  PortDimensions=1
  3x3 Cross Product : aerolibutil/3x3 Cross Product
  CG-CP Transformation : Subsystem
  Demux1 : Demux  Outputs=[3,3]
  Force Transformation : Subsystem
  Moment Transformation : Subsystem
  Mux : Mux  Inputs=3
  Product{,1..3} (4 alike) : Product  SaturateOnIntegerOverflow=on  InputSameDT=on  OutDataTypeStr=Inherit: Same as first input
  Sum : Sum  Inputs=|+-  SaturateOnIntegerOverflow=on
  Sum1 : Sum  Inputs=++|  SaturateOnIntegerOverflow=on  InputSameDT=on  OutDataTypeStr=Inherit: Same as first input
  Vb2 : InportShadow  Port=5
  coefAdjust : Gain  Gain="[-1  1 -1]"
  Forces : Outport  Unit=N
  Moments : Outport  Port=2  Unit=N*m
  wires:
  Vb2/1 -> Moment Transformation/1(Vb)
  Sum1/1 -> Moment Transformation/2(Property-In-Stability (PIS))
  S ref/1 -> Product2/2
  Mux/1 -> Product1/1
  b ref/1 -> Mux/3, Mux/1
  cbar/1 -> Mux/2
  3x3 Cross Product/1 -> Sum1/1
  Product1/1 -> Product3/2
  Coefficients/1 -> Demux1/1
  Demux1/2 -> Product3/1
  qbar/1 -> Product2/1
  Product2/1 -> Product1/2, Product/1
  Product3/1 -> Sum1/2
  Demux1/1 -> coefAdjust/1
  Product/1 -> Force Transformation/2(Property-In-Stability (PIS)), 3x3 Cross Product/1
  Force Transformation/1(Property-In-Body (PIB)) -> Forces/1
  Moment Transformation/1(Property-In-Body (PIB)) -> Moments/1
  coefAdjust/1 -> Product/2
  CG/1 -> Sum/1
  CP/1 -> Sum/2
  Sum/1 -> CG-CP Transformation/2(Property-In-Stability (PIS))
  CG-CP Transformation/1(Property-In-Body (PIB)) -> 3x3 Cross Product/2
  Vb/1 -> Force Transformation/1(Vb), CG-CP Transformation/1(Vb)

== system DatcomForceMoment/Digital DATCOM v1.0.2/Dynamic Contribution/Incidence, Sideslip, & Airspeed1 ==
  Vb : Inport  Unit=m/s
  Airspeed : Sqrt  AlgorithmType=Newton-Raphson  SaturateOnIntegerOverflow=on
  Dot Product : DotProduct  InputSameDT=on  OutDataTypeStr=Inherit: Inherit via internal rule
  Incidence : Trigonometry  Operator=atan2
  Product : Product  Inputs=*/  SaturateOnIntegerOverflow=on  OutDataTypeStr=Inherit: Same as first input
  Selector : Selector  InputPortWidth=3  IndexOptions=Index vector (dialog)  Indices=[2]  OutputSizes=1
  Selector1 : Selector  InputPortWidth=3  IndexOptions=Index vector (dialog)  Indices=[3]  OutputSizes=1
  Selector2 : Selector  InputPortWidth=3  IndexOptions=Index vector (dialog)  Indices=[1]  OutputSizes=1
  Sideslip : Trigonometry  Operator=asin
  Alpha : Outport  Unit=rad  InitialOutput=0
  Beta : Outport  Port=2  Unit=rad  InitialOutput=0
  V : Outport  Port=3  Unit=m/s  InitialOutput=0
  wires:
  Selector/1 -> Product/1
  Sideslip/1 -> Beta/1
  Vb/1 -> Dot Product/2, Dot Product/1, Selector/1, Selector2/1, Selector1/1
  Incidence/1 -> Alpha/1
  Airspeed/1 -> V/1, Product/2
  Dot Product/1 -> Airspeed/1
  Selector2/1 -> Incidence/2
  Selector1/1 -> Incidence/1
  Product/1 -> Sideslip/1

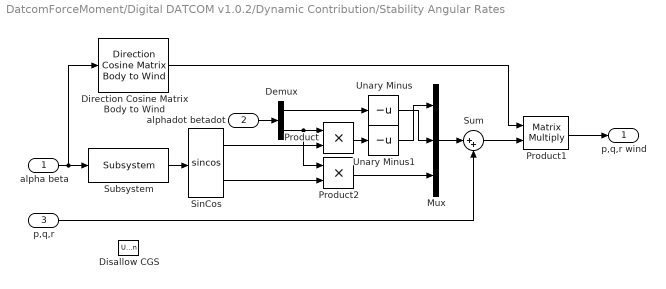
== system DatcomForceMoment/Digital DATCOM v1.0.2/Dynamic Contribution/Stability Angular Rates ==
  alpha beta : Inport  Unit=rad
  alphadot betadot : Inport  Port=2  Unit=rad/s
  p,q,r : Inport  Port=3  Unit=rad/s
  Demux : Demux  Outputs=2
  Direction Cosine Matrix Body to Wind : aerolibtransform2/Direction Cosine Matrix Body to Wind
  Disallow CGS : UnitConfiguration  UnitSystems=DataTag0  UnitSystemsStr=English,SI,SI (extended)  AllowAllUnitSystems=off
  Mux : Mux  Inputs=3
  Product : Product  RndMeth=Zero
  Product1 : Product  Multiplication=Matrix(*)  SaturateOnIntegerOverflow=on  InputSameDT=on  OutDataTypeStr=Inherit: Same as first input
  Product2 : Product  RndMeth=Zero
  SinCos : Trigonometry  Operator=sincos
  Subsystem : aerolibasang/Wind Angular Rates/Subsystem
  Sum : Sum  Inputs=|++
  Unary Minus : UnaryMinus
  Unary Minus1 : UnaryMinus
  p,q,r wind : Outport  Unit=rad/s  InitialOutput=0
  wires:
  alpha beta/1 -> Direction Cosine Matrix Body to Wind/1, Subsystem/1
  Subsystem/1 -> SinCos/1
  SinCos/1 -> Product/2
  SinCos/2 -> Product2/2
  Direction Cosine Matrix Body to Wind/1 -> Product1/1
  Sum/1 -> Product1/2
  Product1/1 -> p,q,r wind/1
  Mux/1 -> Sum/1
  p,q,r/1 -> Sum/2
  alphadot betadot/1 -> Demux/1
  Demux/2 -> Product2/1, Product/1
  Demux/1 -> Unary Minus/1
  Product/1 -> Unary Minus1/1
  Product2/1 -> Mux/3
  Unary Minus1/1 -> Mux/1
  Unary Minus/1 -> Mux/2

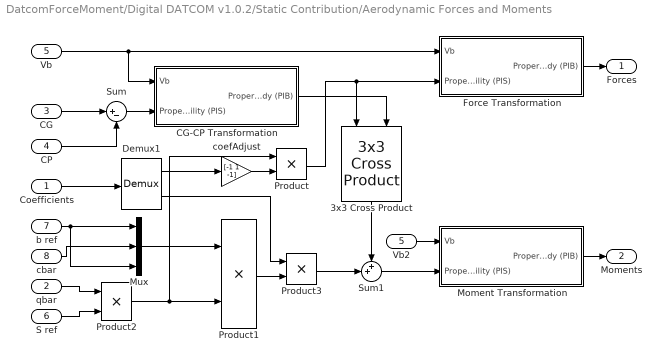
== system DatcomForceMoment/Digital DATCOM v1.0.2/Static Contribution/Aerodynamic Forces and Moments ==
  Coefficients : Inport
  qbar : Inport  Port=2  Unit=Pa
  CG : Inport  Port=3  Unit=m  PortDimensions=[3, 1]
  CP : Inport  Port=4  Unit=m  PortDimensions=[3,1]
  Vb : Inport  Port=5
  S ref : Inport  Port=6  Unit=m^2  PortDimensions=1
  b ref : Inport  Port=7  Unit=m  PortDimensions=1
  cbar : Inport  Port=8  Unit=m  PortDimensions=1
  3x3 Cross Product : aerolibutil/3x3 Cross Product
  CG-CP Transformation : Subsystem
  Demux1 : Demux  Outputs=[3,3]
  Force Transformation : Subsystem
  Moment Transformation : Subsystem
  Mux : Mux  Inputs=3
  Product{,1..3} (4 alike) : Product  SaturateOnIntegerOverflow=on  InputSameDT=on  OutDataTypeStr=Inherit: Same as first input
  Sum : Sum  Inputs=|+-  SaturateOnIntegerOverflow=on
  Sum1 : Sum  Inputs=++|  SaturateOnIntegerOverflow=on  InputSameDT=on  OutDataTypeStr=Inherit: Same as first input
  Vb2 : InportShadow  Port=5
  coefAdjust : Gain  Gain="[-1  1 -1]"
  Forces : Outport  Unit=N
  Moments : Outport  Port=2  Unit=N*m
  wires:
  Vb2/1 -> Moment Transformation/1(Vb)
  Sum1/1 -> Moment Transformation/2(Property-In-Stability (PIS))
  S ref/1 -> Product2/2
  Mux/1 -> Product1/1
  b ref/1 -> Mux/3, Mux/1
  cbar/1 -> Mux/2
  3x3 Cross Product/1 -> Sum1/1
  Product1/1 -> Product3/2
  Coefficients/1 -> Demux1/1
  Demux1/2 -> Product3/1
  qbar/1 -> Product2/1
  Product2/1 -> Product1/2, Product/1
  Product3/1 -> Sum1/2
  Demux1/1 -> coefAdjust/1
  Product/1 -> Force Transformation/2(Property-In-Stability (PIS)), 3x3 Cross Product/1
  Force Transformation/1(Property-In-Body (PIB)) -> Forces/1
  Moment Transformation/1(Property-In-Body (PIB)) -> Moments/1
  coefAdjust/1 -> Product/2
  CG/1 -> Sum/1
  CP/1 -> Sum/2
  Sum/1 -> CG-CP Transformation/2(Property-In-Stability (PIS))
  CG-CP Transformation/1(Property-In-Body (PIB)) -> 3x3 Cross Product/2
  Vb/1 -> Force Transformation/1(Vb), CG-CP Transformation/1(Vb)

== system DatcomForceMoment/Digital DATCOM v1.0.2/Deflection/Aerodynamic Forces and Moments/CG-CP Transformation ==
  Vb : Inport
  Property-In-Stability (PIS) : Inport  Port=2
  Body2Stability : Subsystem
  "Incidence, Sideslip, & Airspeed" : Subsystem
      mask Display:
      | port_label('input',1,'V_b','texmode','on');
      | port_label('output',1,'\alpha','texmode','on');
      | port_label('output',2,'\beta','texmode','on');
      | port_label('output',3,'V','texmode','on');
  Product : Product  Multiplication=Matrix(*)  RndMeth=Zero
  Terminator : Terminator
  Terminator1 : Terminator
  Transpose : Math  Operator=transpose  SaturateOnIntegerOverflow=on
  Property-In-Body (PIB) : Outport
  wires:
  Product/1 -> Property-In-Body (PIB)/1
  Property-In-Stability (PIS)/1 -> Product/2
  "Incidence, Sideslip, & Airspeed"/1(Alpha) -> Body2Stability/1(alpha)
  Body2Stability/1(Ts/b) -> Transpose/1
  Transpose/1 -> Product/1  "Stability2Body"
  Vb/1 -> "Incidence, Sideslip, & Airspeed"/1(Vb)
  "Incidence, Sideslip, & Airspeed"/2(Beta) -> Terminator/1
  "Incidence, Sideslip, & Airspeed"/3(V) -> Terminator1/1

== system DatcomForceMoment/Digital DATCOM v1.0.2/Deflection/Aerodynamic Forces and Moments/Force Transformation ==
  Vb : Inport
  Property-In-Stability (PIS) : Inport  Port=2
  Body2Stability : Subsystem
  "Incidence, Sideslip, & Airspeed" : Subsystem
      mask Display:
      | port_label('input',1,'V_b','texmode','on');
      | port_label('output',1,'\alpha','texmode','on');
      | port_label('output',2,'\beta','texmode','on');
      | port_label('output',3,'V','texmode','on');
  Product : Product  Multiplication=Matrix(*)  RndMeth=Zero
  Terminator : Terminator
  Terminator1 : Terminator
  Transpose : Math  Operator=transpose  SaturateOnIntegerOverflow=on
  Property-In-Body (PIB) : Outport
  wires:
  Product/1 -> Property-In-Body (PIB)/1
  Property-In-Stability (PIS)/1 -> Product/2
  "Incidence, Sideslip, & Airspeed"/1(Alpha) -> Body2Stability/1(alpha)
  Body2Stability/1(Ts/b) -> Transpose/1
  Transpose/1 -> Product/1  "Stability2Body"
  Vb/1 -> "Incidence, Sideslip, & Airspeed"/1(Vb)
  "Incidence, Sideslip, & Airspeed"/2(Beta) -> Terminator/1
  "Incidence, Sideslip, & Airspeed"/3(V) -> Terminator1/1

== system DatcomForceMoment/Digital DATCOM v1.0.2/Deflection/Aerodynamic Forces and Moments/Moment Transformation ==
  Vb : Inport
  Property-In-Stability (PIS) : Inport  Port=2
  Body2Stability : Subsystem
  "Incidence, Sideslip, & Airspeed" : Subsystem
      mask Display:
      | port_label('input',1,'V_b','texmode','on');
      | port_label('output',1,'\alpha','texmode','on');
      | port_label('output',2,'\beta','texmode','on');
      | port_label('output',3,'V','texmode','on');
  Product : Product  Multiplication=Matrix(*)  RndMeth=Zero
  Terminator : Terminator
  Terminator1 : Terminator
  Transpose : Math  Operator=transpose  SaturateOnIntegerOverflow=on
  Property-In-Body (PIB) : Outport
  wires:
  "Incidence, Sideslip, & Airspeed"/3(V) -> Terminator1/1
  "Incidence, Sideslip, & Airspeed"/2(Beta) -> Terminator/1
  Vb/1 -> "Incidence, Sideslip, & Airspeed"/1(Vb)
  Transpose/1 -> Product/1  "Stability2Body"
  Body2Stability/1(Ts/b) -> Transpose/1
  "Incidence, Sideslip, & Airspeed"/1(Alpha) -> Body2Stability/1(alpha)
  Property-In-Stability (PIS)/1 -> Product/2
  Product/1 -> Property-In-Body (PIB)/1

== system DatcomForceMoment/Digital DATCOM v1.0.2/Deflection/Delta Coefficients/Aileron Deflaction ==
  bus : Inport
  Bus Selector : BusSelector  OutputSignals=idxa,fa,idxm,fm,idxh,fh,idxdelta_a,fdelta_a
  Bus Selector1 : BusSelector  OutputSignals=idxa,fa,idxm,fm,idxh,fh,idxdelta_a,fdelta_a
  Constant{1,4..6} (4 alike) : Constant  Value=0
  DCl : Interpolation_n-D  NumberOfTableDimensions=4  Table=permute(datcom.dcl_de,[1 2 3 4])  RemoveProtectionIndex=on
      settings: InputPortMap=u0,u1,u2,u3,u4,u5,u6,u7
  DCn : Interpolation_n-D  NumberOfTableDimensions=4  Table=permute(datcom.dcdi_de,[1 2 3 4])  RemoveProtectionIndex=on
      settings: InputPortMap=u0,u1,u2,u3,u4,u5,u6,u7
  Mux1 : Mux  Inputs=6
  delCoeff_a : Outport
  wires:
  Bus Selector/7 -> DCn/7  "<idxdelta_a>"
  Bus Selector/3 -> DCn/3  "<idxm>"
  Bus Selector1/7 -> DCl/7  "<idxdelta_a>"
  Bus Selector1/3 -> DCl/3  "<idxm>"
  DCl/1 -> Mux1/4  "Cl_a"
  DCn/1 -> Mux1/6  "Cn_a"
  Constant6/1 -> Mux1/1  "CD_a"
  Constant1/1 -> Mux1/2  "CY_a"
  Constant5/1 -> Mux1/3  "CL_e"
  Constant4/1 -> Mux1/5  "Cm_a"
  bus/1 -> Bus Selector/1, Bus Selector1/1
  Bus Selector1/4 -> DCl/4  "<fm>"
  Bus Selector1/6 -> DCl/6  "<fh>"
  Bus Selector1/8 -> DCl/8  "<fdelta_a>"
  Bus Selector1/2 -> DCl/2  "<fa>"
  Bus Selector1/5 -> DCl/5  "<idxh>"
  Bus Selector1/1 -> DCl/1  "<idxa>"
  Mux1/1 -> delCoeff_a/1
  Bus Selector/6 -> DCn/6  "<fh>"
  Bus Selector/8 -> DCn/8  "<fdelta_a>"
  Bus Selector/1 -> DCn/1  "<idxa>"
  Bus Selector/2 -> DCn/2  "<fa>"
  Bus Selector/5 -> DCn/5  "<idxh>"
  Bus Selector/4 -> DCn/4  "<fm>"

== system DatcomForceMoment/Digital DATCOM v1.0.2/Deflection/Delta Coefficients/Elevator Deflaction ==
  bus : Inport
  Bus Selector : BusSelector  OutputSignals=idxa,fa,idxm,fm,idxh,fh,idxd_e,fd_e
  Bus Selector1 : BusSelector  OutputSignals=idxa,fa,idxm,fm,idxh,fh,idxd_e,fd_e
  Bus Selector2 : BusSelector  OutputSignals=idxa,fa,idxm,fm,idxh,fh,idxd_e,fd_e
  Constant1 : Constant  Value=0
  Constant2 : Constant  Value=0
  Constant3 : Constant  Value=0
  DCDI : Interpolation_n-D  NumberOfTableDimensions=4  Table=permute(datcom.dcdi_de,[1 2 3 4])  RemoveProtectionIndex=on
      settings: InputPortMap=u0,u1,u2,u3,u4,u5,u6,u7
  DCL : Interpolation_n-D  NumberOfTableDimensions=4  Table=permute(datcom.dcl_de,[1 2 3 4])  RemoveProtectionIndex=on
      settings: InputPortMap=u0,u1,u2,u3,u4,u5,u6,u7
  DCm : Interpolation_n-D  NumberOfTableDimensions=4  Table=permute(datcom.dcm_de,[1 2 3 4])  RemoveProtectionIndex=on
      settings: InputPortMap=u0,u1,u2,u3,u4,u5,u6,u7
  Mux1 : Mux  Inputs=6
  delCoeff_e : Outport
  wires:
  Bus Selector2/3 -> DCm/3  "<idxm>"
  Bus Selector2/7 -> DCm/7  "<idxd_e>"
  Bus Selector1/7 -> DCL/7  "<idxd_e>"
  Bus Selector1/3 -> DCL/3  "<idxm>"
  Bus Selector/3 -> DCDI/3  "<idxm>"
  Bus Selector/7 -> DCDI/7  "<idxd_e>"
  Constant2/1 -> Mux1/4  "Cl_e"
  Constant3/1 -> Mux1/6  "Cn_e"
  DCDI/1 -> Mux1/1  "CD_e"
  Constant1/1 -> Mux1/2  "CY_e"
  DCL/1 -> Mux1/3  "CL_e"
  DCm/1 -> Mux1/5  "Cm_e"
  Bus Selector/4 -> DCDI/4  "<fm>"
  Bus Selector/5 -> DCDI/5  "<idxh>"
  Bus Selector/2 -> DCDI/2  "<fa>"
  Bus Selector/1 -> DCDI/1  "<idxa>"
  Bus Selector/8 -> DCDI/8  "<fd_e>"
  Bus Selector/6 -> DCDI/6  "<fh>"
  Mux1/1 -> delCoeff_e/1
  Bus Selector1/1 -> DCL/1  "<idxa>"
  Bus Selector1/5 -> DCL/5  "<idxh>"
  Bus Selector1/2 -> DCL/2  "<fa>"
  Bus Selector2/1 -> DCm/1  "<idxa>"
  Bus Selector2/8 -> DCm/8  "<fd_e>"
  Bus Selector2/5 -> DCm/5  "<idxh>"
  Bus Selector2/4 -> DCm/4  "<fm>"
  Bus Selector2/2 -> DCm/2  "<fa>"
  Bus Selector2/6 -> DCm/6  "<fh>"
  Bus Selector1/8 -> DCL/8  "<fd_e>"
  Bus Selector1/6 -> DCL/6  "<fh>"
  Bus Selector1/4 -> DCL/4  "<fm>"
  bus/1 -> Bus Selector/1, Bus Selector1/1, Bus Selector2/1

== system DatcomForceMoment/Digital DATCOM v1.0.2/Deflection/Delta Coefficients/Flap Deflaction ==
  bus : Inport
  Bus Selector : BusSelector  OutputSignals=idxa,fa,idxm,fm,idxh,fh,idxd_f,fd_f
  Bus Selector1 : BusSelector  OutputSignals=idxa,fa,idxm,fm,idxh,fh,idxd_f,fd_f
  Bus Selector4 : BusSelector  OutputSignals=idxa,fa,idxm,fm,idxh,fh,idxd_f,fd_f
  Constant1 : Constant  Value=0
  Constant2 : Constant  Value=0
  Constant3 : Constant  Value=0
  DCDI : Interpolation_n-D  NumberOfTableDimensions=4  Table=permute(datcom.dcdi_df,[1 2 3 4])  RemoveProtectionIndex=on
      settings: InputPortMap=u0,u1,u2,u3,u4,u5,u6,u7
  DCL : Interpolation_n-D  NumberOfTableDimensions=4  Table=permute(datcom.dcl_df,[1 2 3 4])  RemoveProtectionIndex=on
      settings: InputPortMap=u0,u1,u2,u3,u4,u5,u6,u7
  DCm : Interpolation_n-D  NumberOfTableDimensions=4  Table=permute(datcom.dcm_df,[1 2 3 4])  RemoveProtectionIndex=on
      settings: InputPortMap=u0,u1,u2,u3,u4,u5,u6,u7
  Mux1 : Mux  Inputs=6
  delCoeff_f : Outport
  wires:
  Bus Selector4/3 -> DCm/3  "<idxm>"
  Bus Selector4/7 -> DCm/7  "<idxd_f>"
  Bus Selector1/7 -> DCL/7  "<idxd_f>"
  Bus Selector1/3 -> DCL/3  "<idxm>"
  Bus Selector/7 -> DCDI/7  "<idxd_f>"
  Bus Selector/3 -> DCDI/3  "<idxm>"
  Constant2/1 -> Mux1/4  "Cl_f"
  Constant3/1 -> Mux1/6  "Cn_f"
  bus/1 -> Bus Selector1/1, Bus Selector4/1, Bus Selector/1
  Bus Selector1/4 -> DCL/4  "<fm>"
  Bus Selector1/6 -> DCL/6  "<fh>"
  DCDI/1 -> Mux1/1  "CD_f"
  Constant1/1 -> Mux1/2  "CY_f"
  DCL/1 -> Mux1/3  "CL_f"
  Bus Selector1/8 -> DCL/8  "<fd_f>"
  Bus Selector4/6 -> DCm/6  "<fh>"
  Bus Selector4/2 -> DCm/2  "<fa>"
  Bus Selector4/4 -> DCm/4  "<fm>"
  Bus Selector4/5 -> DCm/5  "<idxh>"
  Bus Selector4/8 -> DCm/8  "<fd_f>"
  Bus Selector4/1 -> DCm/1  "<idxa>"
  Bus Selector1/2 -> DCL/2  "<fa>"
  Bus Selector1/5 -> DCL/5  "<idxh>"
  Bus Selector1/1 -> DCL/1  "<idxa>"
  DCm/1 -> Mux1/5  "Cm_f"
  Mux1/1 -> delCoeff_f/1
  Bus Selector/6 -> DCDI/6  "<fh>"
  Bus Selector/8 -> DCDI/8  "<fd_f>"
  Bus Selector/1 -> DCDI/1  "<idxa>"
  Bus Selector/2 -> DCDI/2  "<fa>"
  Bus Selector/5 -> DCDI/5  "<idxh>"
  Bus Selector/4 -> DCDI/4  "<fm>"

== system DatcomForceMoment/Digital DATCOM v1.0.2/Dynamic Contribution/Aerodynamic Forces and Moments Stability Axis/CG-CP Transformation ==
  Vb : Inport
  Property-In-Stability (PIS) : Inport  Port=2
  Body2Stability : Subsystem
  "Incidence, Sideslip, & Airspeed" : Subsystem
      mask Display:
      | port_label('input',1,'V_b','texmode','on');
      | port_label('output',1,'\alpha','texmode','on');
      | port_label('output',2,'\beta','texmode','on');
      | port_label('output',3,'V','texmode','on');
  Product : Product  Multiplication=Matrix(*)  RndMeth=Zero
  Terminator : Terminator
  Terminator1 : Terminator
  Transpose : Math  Operator=transpose  SaturateOnIntegerOverflow=on
  Property-In-Body (PIB) : Outport
  wires:
  Product/1 -> Property-In-Body (PIB)/1
  Property-In-Stability (PIS)/1 -> Product/2
  "Incidence, Sideslip, & Airspeed"/1(Alpha) -> Body2Stability/1(alpha)
  Body2Stability/1(Ts/b) -> Transpose/1
  Transpose/1 -> Product/1  "Stability2Body"
  Vb/1 -> "Incidence, Sideslip, & Airspeed"/1(Vb)
  "Incidence, Sideslip, & Airspeed"/2(Beta) -> Terminator/1
  "Incidence, Sideslip, & Airspeed"/3(V) -> Terminator1/1
